simulink model "TxSteering_RxMVDR_4x4_HDL_IQ"  (R2020a)
settings: Solver=FixedStepDiscrete  StartTime=0.0  StopTime=stoptime*0 + inf  RelTol=1e-3
PreLoadFcn:
  | load('iq_bus_obj.mat');
  | model_init
InitFcn:
  | model_init
model workspace (MAT data in the model file):
  socvcb = containers.Map
  socvcb.serialization.keys = {}
  socvcb.serialization.values = {}
  socvcb.serialization.uniformity = 0
  socvcb.serialization.keyType = 'double'
  socvcb.serialization.valueType = 'any'
values from neighbouring files (symbols this model uses):
  BackSubstitutePrototype = fi(0, matrixdivbacksub_dt)    [model_init.m]
  DataSampleRate = ConverterSampleRate/DecimInterpFactor    (= 245760000)    [model_init.m]
  fc = ConverterSampleRate/4    (= 491520000)    [model_init.m]
  FPGAClkRate = DataSampleRate/VectorSamplingFactor    (= 245760000)    [model_init.m]
  matrixDivDelay = NumberOfCORDICIterations*10 + 86    [model_init.m]
  movavg_bitshift = nextpow2(sqrt(windowSize))    [model_init.m]
  mvdrPipelineDelay = covMatDelay+movAvgDelay+matrixDivDelay+normResponseDelay    [model_init.m]
  NCO_bits = 14    [model_init.m]
  numArrayElements = 4    [model_init.m]
  NumberOfCORDICIterations = matrixdivin_dt.WordLength - 1    [model_init.m]
  S2MM_frame_size = FrameSize*4    (= 40000)    [host_io_init.m]    (also in model_init.m = 1000)
  windowSize = 1024    [model_init.m]
undefined symbols (not defined in the file or in its folder): Fo, Fs, N, physconst
libraries: hdlsllib x268, simulink x53, dspsolvers x1, embreciprocals x1, dsphdlsigops x1
(part 1 of 12)
settings Model: DataTypeOverride=Off  Creator=mfornero  LastModifiedBy=tmealey
settings DataIOCC: SaveOutput=off  SaveTime=off  ReturnWorkspaceOutputs=off
settings OptimizationCC: BlockReduction=off  ConditionallyExecuteInputs=off  DefaultParameterBehavior=Inlined  LifeSpan=inf
settings DebuggingCC: AlgebraicLoopMsg=error  SingleTaskRateTransMsg=error  ParameterPrecisionLossMsg=none  PregeneratedLibrarySubsystemCodeDiagnostic=none  StrictBusMsg=ErrorOnBusTreatedAsVector  SFUnexpectedBacktrackingDiag=warning  SFNoUnconditionalDefaultTransitionDiag=warning  SFExecutionAtInitializationDiag=none  ArithmeticOperatorsInVariantConditions=warning
settings HardwareCC: ProdBitPerPointer=32  ProdBitPerSizeT=32  ProdBitPerPtrDiffT=32  ProdLargestAtomicFloat=None  ProdIntDivRoundTo=Undefined  ProdEndianess=Unspecified  ProdWordSize=32  ProdHWDeviceType=ASIC/FPGA->ASIC/FPGA  ProdEqTarget=off
settings SFSimCC: SimUseLocalCustomCode=off  CustomCodeUndefinedFunction=UseInterfaceOnly
settings RTWCC: RTWUseLocalCustomCode=off
settings CodeAppCC: StateflowObjectComments=on
settings GRTTargetCC: TargetLangStandard=C89/C90 (ANSI)
settings ConfigComp: CovMetricSettings=dw  CovHtmlReporting=on  CovSaveCumulativeToWorkspaceVar=on  CovSaveSingleToWorkspaceVar=on  CovExternalEMLEnable=off

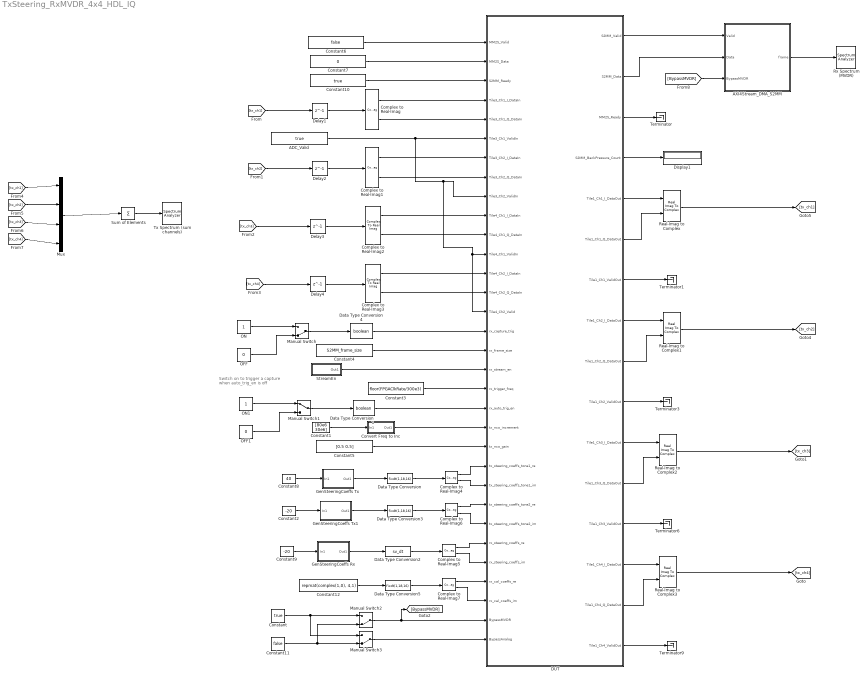
== system TxSteering_RxMVDR_4x4_HDL_IQ ==
  note: Switch on to trigger a capture
      | when auto_trig_en is off
  ADC_Valid : Constant  Value=true  SampleTime=-1
  AXI4Stream_DMA_S2MM : Subsystem
  Complex to Real-Imag{,1..7} (8 alike) : ComplexToRealImag
  Constant : Constant  Value=true  SampleTime=-1
  Constant1 : Constant  Value=[80e6 30e6]  OutDataTypeStr=double  SampleTime=-1
  Constant10 : Constant  Value=true  SampleTime=-1
  Constant11 : Constant  Value=false  SampleTime=-1
  Constant12 : Constant  Value=repmat(complex(1,0), 4,1)  OutDataTypeStr=double  SampleTime=-1
  Constant2 : Constant  Value=-20  OutDataTypeStr=double  SampleTime=-1
  Constant3 : Constant  Value=floor(FPGAClkRate/300e3)  OutDataTypeStr=uint32  SampleTime=-1
  Constant4 : Constant  Value=S2MM_frame_size  OutDataTypeStr=uint32  SampleTime=-1
  Constant5 : Constant  Value=[0.5 0.5]  OutDataTypeStr=fixdt(1,NCO_gain_bits,NCO_gain_bits-1)  SampleTime=-1
  Constant6 : Constant  Value=false  SampleTime=-1
  Constant7 : Constant  Value=0  OutDataTypeStr=fixdt(0,128,0)  SampleTime=-1
  Constant8 : Constant  Value=40  OutDataTypeStr=double  SampleTime=-1
  Constant9 : Constant  Value=-20  OutDataTypeStr=double  SampleTime=-1
  Convert Freq to Inc : Subsystem
  DUT : Subsystem  TreatAsAtomicUnit=on
  Data Type Conversion : DataTypeConversion  OutDataTypeStr=fixdt(1,18,16)
  Data Type Conversion1 : DataTypeConversion  OutDataTypeStr=boolean
  Data Type Conversion2 : DataTypeConversion  OutDataTypeStr=sv_dt
  Data Type Conversion3 : DataTypeConversion  OutDataTypeStr=fixdt(1,18,16)
  Data Type Conversion4 : DataTypeConversion  OutDataTypeStr=boolean
  Data Type Conversion5 : DataTypeConversion  OutDataTypeStr=fixdt(1,18,16)
  Delay{1..4} (4 alike) : Delay  DelayLength=1
  Display1 : Display
  GenSteeringCoeffs Rx : Subsystem
  GenSteeringCoeffs Tx : Subsystem
  GenSteeringCoeffs Tx1 : Subsystem
  Manual Switch : ManualSwitch  CurrentSetting=0
  Manual Switch1 : ManualSwitch
  Manual Switch2 : ManualSwitch  CurrentSetting=0
  Manual Switch3 : ManualSwitch  CurrentSetting=0
  Mux : Mux
  OFF : Constant  Value=0  OutDataTypeStr=boolean  SampleTime=-1
  OFF1 : Constant  Value=0  OutDataTypeStr=boolean  SampleTime=-1
  ON : Constant  OutDataTypeStr=boolean  SampleTime=-1
  ON1 : Constant  OutDataTypeStr=boolean  SampleTime=-1
  Real-Imag to Complex{,1..3} (4 alike) : RealImagToComplex
  Rx Spectrum (MVDR) : SpectrumAnalyzer
  StreamEn : Subsystem
  Sum of Elements : Sum  Inputs=+
  Terminator{,1,3,6,9} (5 alike) : Terminator
  Tx Spectrum (sum channels) : SpectrumAnalyzer
  wires:
  Real-Imag to Complex/1 -> [tx_ch1]
  DUT/2(S2MM_Data) -> AXI4Stream_DMA_S2MM/2(Data)
  Complex to Real-Imag3/2 -> DUT/14(Tile4_Ch2_Q_DataIn)
  Real-Imag to Complex2/1 -> [tx_ch3]
  Complex to Real-Imag4/2 -> DUT/24(tx_steering_coeffs_tone1_im)
  Real-Imag to Complex3/1 -> [tx_ch4]
  Manual Switch3/1 -> DUT/32(BypassAnalog)
  DUT/4(S2MM_BackPressure_Count) -> Display1/1
  Sum of Elements/1 -> Tx Spectrum (sum channels)/1
  Manual Switch2/1 -> [BypassMVDR], DUT/31(BypassMVDR)
  GenSteeringCoeffs Rx/1(Out1) -> Data Type Conversion2/1
  Complex to Real-Imag5/2 -> DUT/28(rx_steering_coeffs_im)
  Real-Imag to Complex1/1 -> [tx_ch2]
  Complex to Real-Imag6/2 -> DUT/26(tx_steering_coeffs_tone2_im)
  Complex to Real-Imag6/1 -> DUT/25(tx_steering_coeffs_tone2_re)
  Complex to Real-Imag5/1 -> DUT/27(rx_steering_coeffs_re)
  Constant2/1 -> GenSteeringCoeffs Tx1/1(In1)
  Convert Freq to Inc/1(Out1) -> DUT/21(tx_nco_increment)
  GenSteeringCoeffs Tx1/1(Out1) -> Data Type Conversion3/1
  Constant7/1 -> DUT/2(MM2S_Data)
  Data Type Conversion3/1 -> Complex to Real-Imag6/1
  [tx_ch4] -> Mux/4
  [tx_ch3] -> Mux/3
  Constant1/1 -> Convert Freq to Inc/1(In1)
  [tx_ch1] -> Mux/1
  [tx_ch2] -> Mux/2
  DUT/7(Tile1_Ch1_ValidOut) -> Terminator1/1
  Mux/1 -> Sum of Elements/1
  AXI4Stream_DMA_S2MM/1(frame) -> Rx Spectrum (MVDR)/1
  DUT/12(Tile1_Ch3_Q_DataOut) -> Real-Imag to Complex2/2
  Constant9/1 -> GenSteeringCoeffs Rx/1(In1)
  Complex to Real-Imag4/1 -> DUT/23(tx_steering_coeffs_tone1_re)
  Data Type Conversion2/1 -> Complex to Real-Imag5/1
  GenSteeringCoeffs Tx/1(Out1) -> Data Type Conversion/1
  Data Type Conversion/1 -> Complex to Real-Imag4/1
  Delay3/1 -> Complex to Real-Imag2/1
  Constant8/1 -> GenSteeringCoeffs Tx/1(In1)
  Constant5/1 -> DUT/22(tx_nco_gain)
  Constant6/1 -> DUT/1(MM2S_Valid)
  DUT/16(Tile1_Ch4_ValidOut) -> Terminator9/1
  Delay4/1 -> Complex to Real-Imag3/1
  [tx_ch4] -> Delay4/1
  Complex to Real-Imag1/1 -> DUT/7(Tile3_Ch2_I_DataIn)
  Complex to Real-Imag3/1 -> DUT/13(Tile4_Ch2_I_DataIn)
  Complex to Real-Imag2/2 -> DUT/11(Tile4_Ch1_Q_DataIn)
  Delay2/1 -> Complex to Real-Imag1/1
  Complex to Real-Imag2/1 -> DUT/10(Tile4_Ch1_I_DataIn)
  [tx_ch3] -> Delay3/1
  [tx_ch2] -> Delay2/1
  Complex to Real-Imag1/2 -> DUT/8(Tile3_Ch2_Q_DataIn)
  [tx_ch1] -> Delay1/1
  DUT/15(Tile1_Ch4_Q_DataOut) -> Real-Imag to Complex3/2
  DUT/14(Tile1_Ch4_I_DataOut) -> Real-Imag to Complex3/1
  DUT/10(Tile1_Ch2_ValidOut) -> Terminator3/1
  DUT/13(Tile1_Ch3_ValidOut) -> Terminator6/1
  DUT/11(Tile1_Ch3_I_DataOut) -> Real-Imag to Complex2/1
  Delay1/1 -> Complex to Real-Imag/1
  DUT/8(Tile1_Ch2_I_DataOut) -> Real-Imag to Complex1/1
  DUT/9(Tile1_Ch2_Q_DataOut) -> Real-Imag to Complex1/2
  DUT/5(Tile1_Ch1_I_DataOut) -> Real-Imag to Complex/1
  DUT/6(Tile1_Ch1_Q_DataOut) -> Real-Imag to Complex/2
  Complex to Real-Imag/2 -> DUT/5(Tile3_Ch1_Q_DataIn)
  Complex to Real-Imag/1 -> DUT/4("Tile3_Ch1_I_DataIn ")
  Constant10/1 -> DUT/3(S2MM_Ready)
  DUT/3(MM2S_Ready) -> Terminator/1
  DUT/1(S2MM_Valid) -> AXI4Stream_DMA_S2MM/1(Valid)
  Manual Switch1/1 -> Data Type Conversion1/1
  ON1/1 -> Manual Switch1/1
  OFF1/1 -> Manual Switch1/2
  Data Type Conversion1/1 -> DUT/20(rx_auto_trig_en)
  Constant3/1 -> DUT/19(rx_trigger_freq)
  StreamEn/1(Out1) -> DUT/18(rx_stream_en)
  OFF/1 -> Manual Switch/2
  ON/1 -> Manual Switch/1
  Manual Switch/1 -> Data Type Conversion4/1
  Constant4/1 -> DUT/17(rx_frame_size)
  Data Type Conversion4/1 -> DUT/16(rx_capture_trig)
  ADC_Valid/1 -> DUT/6(Tile3_Ch1_ValidIn), DUT/15(Tile4_Ch2_Valid), DUT/12(Tile4_Ch1_ValidIn), DUT/9(Tile3_Ch2_ValidIn)
  Constant/1 -> Manual Switch3/1, Manual Switch2/1
  Constant11/1 -> Manual Switch2/2, Manual Switch3/2
  [BypassMVDR] -> AXI4Stream_DMA_S2MM/3(BypassMVDR)
  Data Type Conversion5/1 -> Complex to Real-Imag7/1
  Complex to Real-Imag7/1 -> DUT/29(rx_cal_coeffs_re)
  Complex to Real-Imag7/2 -> DUT/30(rx_cal_coeffs_im)
  Constant12/1 -> Data Type Conversion5/1

== system TxSteering_RxMVDR_4x4_HDL_IQ/AXI4Stream_DMA_S2MM ==
  Valid : Inport
  Data : Inport  Port=2
  BypassMVDR : Inport  Port=3
  Display : Display
  Display1 : Display
  ForCalibration : Subsystem
  HDL Counter : hdlsllib/Sources/HDL Counter  CountType=Free running  CountInit=0  CountStep=1  CountMax=25  CountFromType=Initial value  CountFrom=0  CountResetPort=off  CountLoadPort=off  CountEnbPort=on  CountDirPort=off  CountDataType=Unsigned  CountWordLen=32  CountFracLen=0  CountSampTime=1
  HDL Counter1 : hdlsllib/Sources/HDL Counter  CountType=Free running  CountInit=0  CountStep=1  CountMax=25  CountFromType=Initial value  CountFrom=0  CountResetPort=off  CountLoadPort=off  CountEnbPort=on  CountDirPort=off  CountDataType=Unsigned  CountWordLen=32  CountFracLen=0  CountSampTime=1
  Logical Operator : Logic  AllPortsSameDT=off  OutDataTypeStr=boolean
  ProcessDataFrame : Subsystem
  "S2MM DMA plant " : Subsystem  mask{FRAME_SIZE=S2MM_frame_size}
      mask prompts: FRAME_SIZE "Frame size:"
  frame : Outport
  wires:
  "S2MM DMA plant "/2(frame_valid) -> HDL Counter1/1, Logical Operator/1, ProcessDataFrame/Enable
  Data/1 -> "S2MM DMA plant "/1(data_in)
  Valid/1 -> HDL Counter/1, "S2MM DMA plant "/2(valid_in)
  ProcessDataFrame/1(Out1) -> frame/1
  BypassMVDR/1 -> Logical Operator/2
  Logical Operator/1 -> ForCalibration/Enable
  "S2MM DMA plant "/1(frame_data) -> ProcessDataFrame/1(In1), ForCalibration/1(In1)
  HDL Counter/1 -> Display/1
  HDL Counter1/1 -> Display1/1

== system TxSteering_RxMVDR_4x4_HDL_IQ/Convert Freq to Inc ==
  In1 : Inport
  Data Type Conversion : DataTypeConversion  OutDataTypeStr=fixdt(0,NCO_bits,0)
  Floor : Rounding
  Gain : Gain  Gain=2^NCO_bits/DataSampleRate
  Out1 : Outport
  wires:
  In1/1 -> Gain/1
  Gain/1 -> Floor/1
  Floor/1 -> Data Type Conversion/1
  Data Type Conversion/1 -> Out1/1

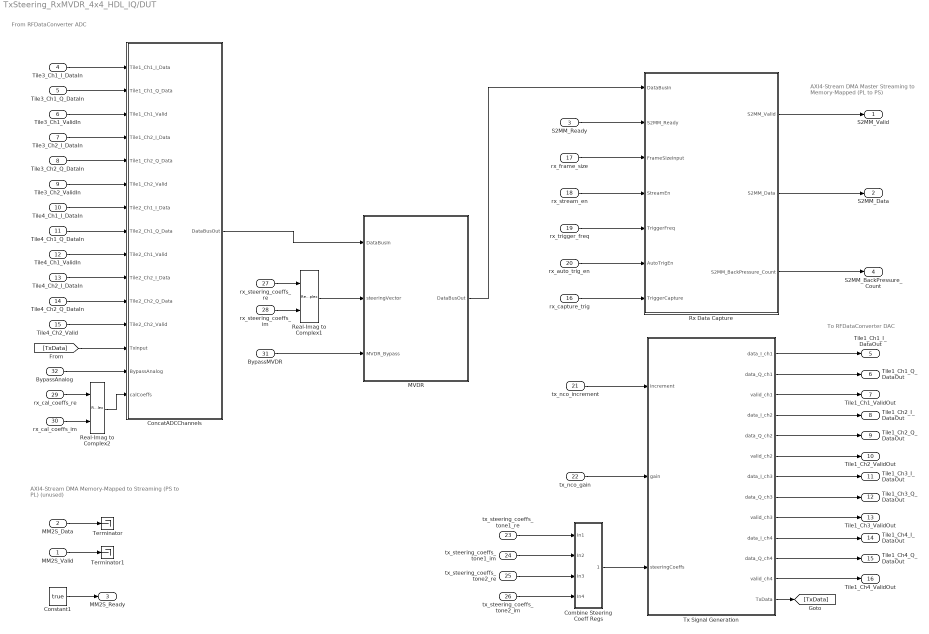
== system TxSteering_RxMVDR_4x4_HDL_IQ/DUT ==
  note: AXI4-Stream DMA Master
      | Streaming to Memory-Mapped (PL to PS)
  note: AXI4-Stream DMA
      | Memory-Mapped to Streaming (PS to PL)
      | (unused)
  note: From RFDataConverter ADC
  note: To RFDataConverter DAC
  MM2S_Valid : Inport
  MM2S_Data : Inport  Port=2
  S2MM_Ready : Inport  Port=3
  "Tile3_Ch1_I_DataIn " : Inport  Port=4
  Tile3_Ch1_Q_DataIn : Inport  Port=5
  Tile3_Ch1_ValidIn : Inport  Port=6
  Tile3_Ch2_I_DataIn : Inport  Port=7
  Tile3_Ch2_Q_DataIn : Inport  Port=8
  Tile3_Ch2_ValidIn : Inport  Port=9
  Tile4_Ch1_I_DataIn : Inport  Port=10
  Tile4_Ch1_Q_DataIn : Inport  Port=11
  Tile4_Ch1_ValidIn : Inport  Port=12
  Tile4_Ch2_I_DataIn : Inport  Port=13
  Tile4_Ch2_Q_DataIn : Inport  Port=14
  Tile4_Ch2_Valid : Inport  Port=15
  rx_capture_trig : Inport  Port=16
  rx_frame_size : Inport  Port=17
  rx_stream_en : Inport  Port=18
  rx_trigger_freq : Inport  Port=19
  rx_auto_trig_en : Inport  Port=20
  tx_nco_increment : Inport  Port=21  OutDataTypeStr=fixdt(0,NCO_bits,0)
  tx_nco_gain : Inport  Port=22  OutDataTypeStr=fixdt(1,NCO_gain_bits,NCO_gain_bits-1)
  tx_steering_coeffs_tone1_re : Inport  Port=23  PortDimensions=NumChan
  tx_steering_coeffs_tone1_im : Inport  Port=24  PortDimensions=NumChan
  tx_steering_coeffs_tone2_re : Inport  Port=25  PortDimensions=NumChan
  tx_steering_coeffs_tone2_im : Inport  Port=26  PortDimensions=NumChan
  rx_steering_coeffs_re : Inport  Port=27  PortDimensions=NumChan
  rx_steering_coeffs_im : Inport  Port=28  PortDimensions=NumChan
  rx_cal_coeffs_re : Inport  Port=29  PortDimensions=NumChan
  rx_cal_coeffs_im : Inport  Port=30  PortDimensions=NumChan
  BypassMVDR : Inport  Port=31
  BypassAnalog : Inport  Port=32
  Combine Steering Coeff Regs : Subsystem
  ConcatADCChannels : Subsystem
  Constant1 : Constant  Value=true  OutDataTypeStr=boolean  SampleTime=-1
  MVDR : Subsystem
  Real-Imag to Complex1 : RealImagToComplex
  Real-Imag to Complex2 : RealImagToComplex
  Rx Data Capture : Subsystem
  Terminator : Terminator
  Terminator1 : Terminator
  Tx Signal Generation : Subsystem
  S2MM_Valid : Outport  VectorParamsAs1DForOutWhenUnconnected=off
  S2MM_Data : Outport  Port=2  VectorParamsAs1DForOutWhenUnconnected=off
  MM2S_Ready : Outport  Port=3  VectorParamsAs1DForOutWhenUnconnected=off
  S2MM_BackPressure_Count : Outport  Port=4  VectorParamsAs1DForOutWhenUnconnected=off
  Tile1_Ch1_I_DataOut : Outport  Port=5  VectorParamsAs1DForOutWhenUnconnected=off
  Tile1_Ch1_Q_DataOut : Outport  Port=6  VectorParamsAs1DForOutWhenUnconnected=off
  Tile1_Ch1_ValidOut : Outport  Port=7  VectorParamsAs1DForOutWhenUnconnected=off
  Tile1_Ch2_I_DataOut : Outport  Port=8  VectorParamsAs1DForOutWhenUnconnected=off
  Tile1_Ch2_Q_DataOut : Outport  Port=9  VectorParamsAs1DForOutWhenUnconnected=off
  Tile1_Ch2_ValidOut : Outport  Port=10  VectorParamsAs1DForOutWhenUnconnected=off
  Tile1_Ch3_I_DataOut : Outport  Port=11  VectorParamsAs1DForOutWhenUnconnected=off
  Tile1_Ch3_Q_DataOut : Outport  Port=12  VectorParamsAs1DForOutWhenUnconnected=off
  Tile1_Ch3_ValidOut : Outport  Port=13  VectorParamsAs1DForOutWhenUnconnected=off
  Tile1_Ch4_I_DataOut : Outport  Port=14  VectorParamsAs1DForOutWhenUnconnected=off
  Tile1_Ch4_Q_DataOut : Outport  Port=15  VectorParamsAs1DForOutWhenUnconnected=off
  Tile1_Ch4_ValidOut : Outport  Port=16  VectorParamsAs1DForOutWhenUnconnected=off
  wires:
  Constant1/1 -> MM2S_Ready/1
  S2MM_Ready/1 -> Rx Data Capture/2(S2MM_Ready)
  rx_frame_size/1 -> Rx Data Capture/3(FrameSizeInput)
  rx_stream_en/1 -> Rx Data Capture/4(StreamEn)
  rx_trigger_freq/1 -> Rx Data Capture/5(TriggerFreq)
  rx_auto_trig_en/1 -> Rx Data Capture/6(AutoTrigEn)
  rx_capture_trig/1 -> Rx Data Capture/7(TriggerCapture)
  Rx Data Capture/1(S2MM_Valid) -> S2MM_Valid/1
  Rx Data Capture/2(S2MM_Data) -> S2MM_Data/1
  Rx Data Capture/3(S2MM_BackPressure_Count) -> S2MM_BackPressure_Count/1
  "Tile3_Ch1_I_DataIn "/1 -> ConcatADCChannels/1("Tile1_Ch1_I_Data ")
  Tile3_Ch1_ValidIn/1 -> ConcatADCChannels/3(Tile1_Ch1_Valid)
  Tile3_Ch1_Q_DataIn/1 -> ConcatADCChannels/2(Tile1_Ch1_Q_Data)
  Tile3_Ch2_I_DataIn/1 -> ConcatADCChannels/4(Tile1_Ch2_I_Data)
  Tile3_Ch2_ValidIn/1 -> ConcatADCChannels/6(Tile1_Ch2_Valid)
  Tile3_Ch2_Q_DataIn/1 -> ConcatADCChannels/5(Tile1_Ch2_Q_Data)
  Tile4_Ch1_I_DataIn/1 -> ConcatADCChannels/7(Tile2_Ch1_I_Data)
  Tile4_Ch1_ValidIn/1 -> ConcatADCChannels/9(Tile2_Ch1_Valid)
  Tile4_Ch1_Q_DataIn/1 -> ConcatADCChannels/8(Tile2_Ch1_Q_Data)
  Tile4_Ch2_I_DataIn/1 -> ConcatADCChannels/10(Tile2_Ch2_I_Data)
  Tile4_Ch2_Valid/1 -> ConcatADCChannels/12(Tile2_Ch2_Valid)
  Tile4_Ch2_Q_DataIn/1 -> ConcatADCChannels/11(Tile2_Ch2_Q_Data)
  MM2S_Data/1 -> Terminator/1
  MM2S_Valid/1 -> Terminator1/1
  Tx Signal Generation/1(data_I_ch1) -> Tile1_Ch1_I_DataOut/1
  Tx Signal Generation/2(data_Q_ch1) -> Tile1_Ch1_Q_DataOut/1
  tx_nco_increment/1 -> Tx Signal Generation/1(increment)
  tx_nco_gain/1 -> Tx Signal Generation/2(gain)
  Tx Signal Generation/3(valid_ch1) -> Tile1_Ch1_ValidOut/1
  Tx Signal Generation/4(data_I_ch2) -> Tile1_Ch2_I_DataOut/1
  Tx Signal Generation/5(data_Q_ch2) -> Tile1_Ch2_Q_DataOut/1
  Tx Signal Generation/6(valid_ch2) -> Tile1_Ch2_ValidOut/1
  Tx Signal Generation/7(data_I_ch3) -> Tile1_Ch3_I_DataOut/1
  Tx Signal Generation/8(data_Q_ch3) -> Tile1_Ch3_Q_DataOut/1
  Tx Signal Generation/9(valid_ch3) -> Tile1_Ch3_ValidOut/1
  Tx Signal Generation/10(data_I_ch4) -> Tile1_Ch4_I_DataOut/1
  Tx Signal Generation/11(data_Q_ch4) -> Tile1_Ch4_Q_DataOut/1
  Tx Signal Generation/12(valid_ch4) -> Tile1_Ch4_ValidOut/1
  rx_steering_coeffs_im/1 -> Real-Imag to Complex1/2
  Real-Imag to Complex1/1 -> MVDR/2(steeringVector)
  rx_steering_coeffs_re/1 -> Real-Imag to Complex1/1
  ConcatADCChannels/1(DataBusOut) -> MVDR/1(DataBusIn)
  tx_steering_coeffs_tone1_re/1 -> Combine Steering Coeff Regs/1(In1)
  tx_steering_coeffs_tone1_im/1 -> Combine Steering Coeff Regs/2(In2)
  tx_steering_coeffs_tone2_re/1 -> Combine Steering Coeff Regs/3(In3)
  tx_steering_coeffs_tone2_im/1 -> Combine Steering Coeff Regs/4(In4)
  Combine Steering Coeff Regs/1(Out1) -> Tx Signal Generation/3(steeringCoeffs)
  MVDR/1(DataBusOut) -> Rx Data Capture/1(DataBusIn)
  Tx Signal Generation/13(TxData) -> [TxData]
  [TxData] -> ConcatADCChannels/13(TxInput)
  BypassMVDR/1 -> MVDR/3(MVDR_Bypass)
  BypassAnalog/1 -> ConcatADCChannels/14(BypassAnalog)
  rx_cal_coeffs_re/1 -> Real-Imag to Complex2/1
  rx_cal_coeffs_im/1 -> Real-Imag to Complex2/2
  Real-Imag to Complex2/1 -> ConcatADCChannels/15(calCoeffs)

== system TxSteering_RxMVDR_4x4_HDL_IQ/GenSteeringCoeffs Rx ==
  In1 : Inport
  Constant : Constant  Value=fc  SampleTime=-1
  Constant9 : Constant  Value=0  OutDataTypeStr=double  SampleTime=-1
  MATLAB System1 : MATLABSystem  System=phased.SteeringVector  PropagationSpeed=physconst( 'LightSpeed' )  IncludeElementResponse=off  NumPhaseShifterBits=0  EnablePolarization=off  SimulateUsing=Interpreted execution  SensorArray=sensorArray
      mask Type: phased.SteeringVector
      mask Display:
      | disp(['Steering' char(10) 'Vector']);
      | port_label('input',1,'Freq');
      | port_label('input',2,'Ang');
  Vector Concatenate : Concatenate  Mode=Multidimensional array
  Out1 : Outport
  wires:
  Vector Concatenate/1 -> MATLAB System1/2
  Constant/1 -> MATLAB System1/1
  In1/1 -> Vector Concatenate/1
  Constant9/1 -> Vector Concatenate/2
  MATLAB System1/1 -> Out1/1

== system TxSteering_RxMVDR_4x4_HDL_IQ/GenSteeringCoeffs Tx ==
  In1 : Inport
  Constant : Constant  Value=fc  SampleTime=-1
  Constant9 : Constant  Value=0  OutDataTypeStr=double  SampleTime=-1
  MATLAB System1 : MATLABSystem  System=phased.SteeringVector  PropagationSpeed=physconst( 'LightSpeed' )  IncludeElementResponse=off  NumPhaseShifterBits=0  EnablePolarization=off  SimulateUsing=Interpreted execution  SensorArray=sensorArray
      mask Type: phased.SteeringVector
      mask Display:
      | disp(['Steering' char(10) 'Vector']);
      | port_label('input',1,'Freq');
      | port_label('input',2,'Ang');
  Vector Concatenate : Concatenate  Mode=Multidimensional array
  Out1 : Outport
  wires:
  MATLAB System1/1 -> Out1/1
  Constant9/1 -> Vector Concatenate/2
  In1/1 -> Vector Concatenate/1
  Constant/1 -> MATLAB System1/1
  Vector Concatenate/1 -> MATLAB System1/2

== system TxSteering_RxMVDR_4x4_HDL_IQ/GenSteeringCoeffs Tx1 ==
  In1 : Inport
  Constant : Constant  Value=fc  SampleTime=-1
  Constant9 : Constant  Value=0  OutDataTypeStr=double  SampleTime=-1
  MATLAB System1 : MATLABSystem  System=phased.SteeringVector  PropagationSpeed=physconst( 'LightSpeed' )  IncludeElementResponse=off  NumPhaseShifterBits=0  EnablePolarization=off  SimulateUsing=Interpreted execution  SensorArray=sensorArray
      mask Type: phased.SteeringVector
      mask Display:
      | disp(['Steering' char(10) 'Vector']);
      | port_label('input',1,'Freq');
      | port_label('input',2,'Ang');
  Vector Concatenate : Concatenate  Mode=Multidimensional array
  Out1 : Outport
  wires:
  Vector Concatenate/1 -> MATLAB System1/2
  Constant/1 -> MATLAB System1/1
  In1/1 -> Vector Concatenate/1
  Constant9/1 -> Vector Concatenate/2
  MATLAB System1/1 -> Out1/1

== system TxSteering_RxMVDR_4x4_HDL_IQ/StreamEn ==
  Data Type Conversion1 : DataTypeConversion  OutDataTypeStr=boolean
  Manual Switch1 : ManualSwitch
  OFF : Constant  Value=0  OutDataTypeStr=boolean  SampleTime=-1
  ON : Constant  OutDataTypeStr=boolean  SampleTime=-1
  Out1 : Outport  VectorParamsAs1DForOutWhenUnconnected=off
  wires:
  Data Type Conversion1/1 -> Out1/1
  OFF/1 -> Manual Switch1/2
  ON/1 -> Manual Switch1/1
  Manual Switch1/1 -> Data Type Conversion1/1

== system TxSteering_RxMVDR_4x4_HDL_IQ/AXI4Stream_DMA_S2MM/ForCalibration ==
  In1 : Inport
  Enable : EnablePort
  Rx Spectrum (MVDR) : SpectrumAnalyzer
  Selector : Selector  NumberOfDimensions=2  InputPortWidth=3  IndexOptions=Select all,Index vector (dialog)  Indices=[1 3],1  OutputSizes=1,1
  Selector1 : Selector  NumberOfDimensions=2  InputPortWidth=3  IndexOptions=Select all,Index vector (dialog)  Indices=[1 3],2  OutputSizes=1,1
  Selector2 : Selector  NumberOfDimensions=2  InputPortWidth=3  IndexOptions=Select all,Index vector (dialog)  Indices=[1 3],3  OutputSizes=1,1
  Selector3 : Selector  NumberOfDimensions=2  InputPortWidth=3  IndexOptions=Select all,Index vector (dialog)  Indices=[1 3],4  OutputSizes=1,1
  Time Scope : Scope  NumInputPorts=4
  Unpack Complex : Subsystem
  wires:
  In1/1 -> Unpack Complex/1(In1)
  Unpack Complex/1(Out1) -> Selector3/1, Selector2/1, Selector1/1, Selector/1
  Selector1/1 -> Time Scope/2
  Selector/1 -> Time Scope/1
  Selector2/1 -> Time Scope/3
  Selector3/1 -> Rx Spectrum (MVDR)/1, Time Scope/4

== system TxSteering_RxMVDR_4x4_HDL_IQ/AXI4Stream_DMA_S2MM/ProcessDataFrame ==
  In1 : Inport
  Enable : EnablePort
  Data Type Conversion5 : DataTypeConversion  OutDataTypeStr=fixdt(1,64,0)  ConvertRealWorld=Stored Integer (SI)
  Unpack Complex : Subsystem
  Out1 : Outport
  wires:
  In1/1 -> Data Type Conversion5/1
  Unpack Complex/1(Out1) -> Out1/1
  Data Type Conversion5/1 -> Unpack Complex/1(In1)

== system TxSteering_RxMVDR_4x4_HDL_IQ/AXI4Stream_DMA_S2MM/S2MM DMA plant  ==
  data_in : Inport
  valid_in : Inport  Port=2
  MATLAB Function1 : MATLAB Function  TreatAsAtomicUnit=on
  frame_data : Outport
  frame_valid : Outport  Port=2
  wires:
  valid_in/1 -> MATLAB Function1/2(valid_i)
  MATLAB Function1/1(data_o) -> frame_data/1
  MATLAB Function1/2(valid_o) -> frame_valid/1
  data_in/1 -> MATLAB Function1/1(data_i)

== system TxSteering_RxMVDR_4x4_HDL_IQ/DUT/Combine Steering Coeff Regs ==
  In1 : Inport
  In2 : Inport  Port=2
  In3 : Inport  Port=3
  In4 : Inport  Port=4
  Real-Imag to Complex : RealImagToComplex
  Real-Imag to Complex2 : RealImagToComplex
  Vector Concatenate : Concatenate
  Out1 : Outport
  wires:
  In1/1 -> Real-Imag to Complex/1
  In2/1 -> Real-Imag to Complex/2
  In4/1 -> Real-Imag to Complex2/2
  In3/1 -> Real-Imag to Complex2/1
  Real-Imag to Complex/1 -> Vector Concatenate/1
  Real-Imag to Complex2/1 -> Vector Concatenate/2
  Vector Concatenate/1 -> Out1/1

== system TxSteering_RxMVDR_4x4_HDL_IQ/DUT/ConcatADCChannels ==
  "Tile1_Ch1_I_Data " : Inport
  Tile1_Ch1_Q_Data : Inport  Port=2
  Tile1_Ch1_Valid : Inport  Port=3
  Tile1_Ch2_I_Data : Inport  Port=4
  Tile1_Ch2_Q_Data : Inport  Port=5
  Tile1_Ch2_Valid : Inport  Port=6
  Tile2_Ch1_I_Data : Inport  Port=7
  Tile2_Ch1_Q_Data : Inport  Port=8
  Tile2_Ch1_Valid : Inport  Port=9
  Tile2_Ch2_I_Data : Inport  Port=10
  Tile2_Ch2_Q_Data : Inport  Port=11
  Tile2_Ch2_Valid : Inport  Port=12
  TxInput : Inport  Port=13
  BypassAnalog : Inport  Port=14
  calCoeffs : Inport  Port=15
  Apply Calibration Coefficients : Subsystem
  Data Type Conversion : DataTypeConversion  OutDataTypeStr=input_dt  ConvertRealWorld=Stored Integer (SI)
  Delay1 : Delay  DelayLength=1
  Delay2 : Delay  DelayLength=1
  Real-Imag to Complex{,1..3} (4 alike) : RealImagToComplex
  Switch : Switch  Criteria=u2 > Threshold
  Terminator : Terminator
  Terminator3 : Terminator
  Terminator5 : Terminator
  To Data Bus : Subsystem  mask(To Data Bus){dummy=0}
      mask help: Create a streaming Data Bus from Data and Valid signals.
      mask Display:
      | port_label('input',1,'data');
      | port_label('input',2,'valid');
  Vector Concatenate : Concatenate  NumInputs=4  Mode=Multidimensional array  ConcatenateDimension=2
  DataBusOut : Outport  VectorParamsAs1DForOutWhenUnconnected=off
  wires:
  Tile1_Ch2_Valid/1 -> Terminator/1
  Tile2_Ch1_Valid/1 -> Terminator3/1
  Tile2_Ch2_Valid/1 -> Terminator5/1
  Real-Imag to Complex/1 -> Vector Concatenate/1
  Real-Imag to Complex1/1 -> Vector Concatenate/2
  Real-Imag to Complex2/1 -> Vector Concatenate/3
  Real-Imag to Complex3/1 -> Vector Concatenate/4
  Vector Concatenate/1 -> Data Type Conversion/1
  To Data Bus/1(bus) -> Delay2/1
  "Tile1_Ch1_I_Data "/1 -> Real-Imag to Complex/1
  Tile1_Ch1_Q_Data/1 -> Real-Imag to Complex/2
  Tile1_Ch2_I_Data/1 -> Real-Imag to Complex1/1
  Tile1_Ch2_Q_Data/1 -> Real-Imag to Complex1/2
  Tile2_Ch1_I_Data/1 -> Real-Imag to Complex2/1
  Tile2_Ch1_Q_Data/1 -> Real-Imag to Complex2/2
  Tile2_Ch2_I_Data/1 -> Real-Imag to Complex3/1
  Tile2_Ch2_Q_Data/1 -> Real-Imag to Complex3/2
  TxInput/1 -> Switch/1
  Switch/1 -> Delay1/1
  BypassAnalog/1 -> Switch/2
  Delay1/1 -> DataBusOut/1
  Delay2/1 -> Switch/3
  Data Type Conversion/1 -> Apply Calibration Coefficients/1(dataIn)
  Apply Calibration Coefficients/1(dataOut) -> To Data Bus/1(data)
  Apply Calibration Coefficients/2(validOut) -> To Data Bus/2(valid)
  calCoeffs/1 -> Apply Calibration Coefficients/3(coeffIn)
  Tile1_Ch1_Valid/1 -> Apply Calibration Coefficients/2(validIn)

== system TxSteering_RxMVDR_4x4_HDL_IQ/DUT/MVDR ==
  DataBusIn : Inport
  steeringVector : Inport  Port=2
  MVDR_Bypass : Inport  Port=3
  Compute Weight Vector : Subsystem
  Delay5 : Delay  DelayLength=mvdrPipelineDelay
  Form Beam : Subsystem
  Form Covariance Matrix : Subsystem
  From Data Bus : Subsystem  mask(From Data Bus){dummy=0}
      mask help: Convert a streaming Data Bus to individual Data and Valid signals.
      mask Display:
      | port_label('output',1,'data');
      | port_label('output',2,'valid');
  Moving Average : Subsystem
  Normalize Response : Subsystem
  Subsystem : Subsystem
  DataBusOut : Outport
  wires:
  Form Covariance Matrix/2(validOut) -> Moving Average/2(validIn)
  Compute Weight Vector/1(w) -> Normalize Response/1(wIn)
  steeringVector/1 -> Normalize Response/3(steeringVector), Compute Weight Vector/3(steeringVector)
  Form Covariance Matrix/1(dataOut) -> Moving Average/1(dataIn)
  DataBusIn/1 -> Delay5/1, Subsystem/2(Bypass_Input), From Data Bus/1(bus)
  Moving Average/1(dataOut) -> Compute Weight Vector/1(covarianceMatrix)
  Delay5/1 -> Form Beam/1(DataBusIn)
  Moving Average/2(validOut) -> Compute Weight Vector/2(validIn)
  From Data Bus/2(valid) -> Form Covariance Matrix/2(validIn)
  From Data Bus/1(data) -> Form Covariance Matrix/1(dataIn)
  Form Beam/1(DataBusOut) -> Subsystem/3(MVDR_Input)
  Subsystem/1(DataOut) -> DataBusOut/1
  MVDR_Bypass/1 -> Subsystem/1(BypassEn)
  Compute Weight Vector/2(validOut) -> Normalize Response/2(validIn)
  Normalize Response/1(wOut) -> Form Beam/2(w)

== system TxSteering_RxMVDR_4x4_HDL_IQ/DUT/Rx Data Capture ==
  Bus Element In : Inport  PortName=DataBusIn  Element=data
  Bus Element In1 : Inport  PortName=DataBusIn  Element=valid
  S2MM_Ready : Inport  Port=2
  FrameSizeInput : Inport  Port=3
  StreamEn : Inport  Port=4
  TriggerFreq : Inport  Port=5
  AutoTrigEn : Inport  Port=6
  TriggerCapture : Inport  Port=7
  AXI4-Lite Initial Value : Subsystem  mask(AXI4-Lite Initial Value){x0=uint32(floor(FPGAClkRate/2))}
      mask prompts: x0 "Initial value:"
      mask help: Set the initial value for an AXI4-Lite register.
      mask Display: fprintf('x0 = %g',x0);
  AutoTrigger : Subsystem
  Delay{2,4..6,25..26} (6 alike) : Delay  DelayLength=1
  EnableConsecutiveFrames : Subsystem
  HDL Counter : hdlsllib/Sources/HDL Counter  CountType=Free running  CountInit=0  CountStep=1  CountMax=25  CountFromType=Initial value  CountFrom=0  CountResetPort=off  CountLoadPort=off  CountEnbPort=on  CountDirPort=off  CountDataType=Unsigned  CountWordLen=32  CountFracLen=0  CountSampTime=1
  Logical Operator6 : Logic  Operator=NOT  IconShape=distinctive  AllPortsSameDT=off  OutDataTypeStr=boolean
  Signal Specification : SignalSpecification  SampleTime=1/FPGAClkRate
  "Stream FIFO " : Subsystem
  Switch : Switch  Criteria=u2 > Threshold
  Terminator : Terminator
  Terminator3 : Terminator
  S2MM_Valid : Outport  VectorParamsAs1DForOutWhenUnconnected=off
  S2MM_Data : Outport  Port=2  VectorParamsAs1DForOutWhenUnconnected=off
  S2MM_BackPressure_Count : Outport  Port=3  VectorParamsAs1DForOutWhenUnconnected=off
  wires:
  S2MM_Ready/1 -> Delay4/1
  Delay6/1 -> AutoTrigger/2(SW_en), "Stream FIFO "/5(StreamEn)
  Delay26/1 -> "Stream FIFO "/3(TValid)
  AutoTrigger/1(Trig) -> Switch/1  "Trig"
  TriggerCapture/1 -> Delay5/1
  FrameSizeInput/1 -> Delay2/1
  Delay4/1 -> "Stream FIFO "/1(TReady)
  StreamEn/1 -> Delay6/1
  Delay5/1 -> Switch/3
  "Stream FIFO "/5(AFull) -> HDL Counter/1, Logical Operator6/1  "AlmostFull"
  "Stream FIFO "/2(ValidOut) -> S2MM_Valid/1
  EnableConsecutiveFrames/1(DataCaptureEn) -> "Stream FIFO "/4(TriggerCapture)
  "Stream FIFO "/4(Full) -> Terminator3/1
  Logical Operator6/1 -> EnableConsecutiveFrames/3(BackPressureCounterEn)
  TriggerFreq/1 -> AXI4-Lite Initial Value/1(In1)
  AXI4-Lite Initial Value/1(Out1) -> AutoTrigger/1(MaxCount)
  "Stream FIFO "/3(Num) -> Terminator/1
  AutoTrigEn/1 -> Switch/2
  Delay25/1 -> Signal Specification/1
  Delay2/1 -> EnableConsecutiveFrames/2(ConsecFrames)
  Switch/1 -> EnableConsecutiveFrames/1(Trigger)  "TriggerInput"
  HDL Counter/1 -> S2MM_BackPressure_Count/1
  "Stream FIFO "/1(TDataOut) -> S2MM_Data/1
  Bus Element In1/1 -> Delay26/1
  Signal Specification/1 -> "Stream FIFO "/2(TData)
  Bus Element In/1 -> Delay25/1

== system TxSteering_RxMVDR_4x4_HDL_IQ/DUT/Tx Signal Generation ==
  increment : Inport
  gain : Inport  Port=2
  steeringCoeffs : Inport  Port=3
  Combine Channels : Subsystem
  Complex to Real-Imag : ComplexToRealImag
  ConcatADCChannels : Subsystem
  Delay : Delay  DelayLength=1
  Demux : Demux
  Demux1 : Demux
  Generate Steering Channels : Subsystem  TreatAsAtomicUnit=on
  data_I_ch1 : Outport
  data_Q_ch1 : Outport  Port=2
  valid_ch1 : Outport  Port=3
  data_I_ch2 : Outport  Port=4
  data_Q_ch2 : Outport  Port=5
  valid_ch2 : Outport  Port=6
  data_I_ch3 : Outport  Port=7
  data_Q_ch3 : Outport  Port=8
  valid_ch3 : Outport  Port=9
  data_I_ch4 : Outport  Port=10
  data_Q_ch4 : Outport  Port=11
  valid_ch4 : Outport  Port=12
  TxData : Outport  Port=13
  wires:
  Demux/1 -> data_I_ch1/1, ConcatADCChannels/1("Tile1_Ch1_I_Data ")
  Demux/4 -> data_I_ch4/1, ConcatADCChannels/7(Tile2_Ch2_I_Data)
  Demux/3 -> data_I_ch3/1, ConcatADCChannels/5(Tile2_Ch1_I_Data)
  Demux/2 -> ConcatADCChannels/3(Tile1_Ch2_I_Data), data_I_ch2/1
  Demux1/1 -> ConcatADCChannels/2(Tile1_Ch1_Q_Data), data_Q_ch1/1
  Demux1/2 -> ConcatADCChannels/4(Tile1_Ch2_Q_Data), data_Q_ch2/1
  Demux1/3 -> ConcatADCChannels/6(Tile2_Ch1_Q_Data), data_Q_ch3/1
  Demux1/4 -> ConcatADCChannels/8(Tile2_Ch2_Q_Data), data_Q_ch4/1
  Complex to Real-Imag/2 -> Demux1/1
  Complex to Real-Imag/1 -> Demux/1
  increment/1 -> Generate Steering Channels/1(increment)
  gain/1 -> Generate Steering Channels/2(gain)
  steeringCoeffs/1 -> Generate Steering Channels/3(steeringCoeffs)
  Combine Channels/2(validOut) -> ConcatADCChannels/9(Valid), valid_ch1/1, valid_ch4/1, valid_ch3/1, valid_ch2/1
  Generate Steering Channels/1(dataOut) -> Combine Channels/1(dataIn)
  Generate Steering Channels/2(validOut) -> Combine Channels/2(validIn)
  Combine Channels/1(dataOut) -> Complex to Real-Imag/1
  ConcatADCChannels/1(DataBusOut) -> Delay/1
  Delay/1 -> TxData/1

== system TxSteering_RxMVDR_4x4_HDL_IQ/AXI4Stream_DMA_S2MM/ForCalibration/Unpack Complex ==
  In1 : Inport
  Extract Bits2 : simulink/Logic and Bit Operations/Extract Bits  bitsToExtract=Lower half  numBits=8  bitIdxRange=[0 7]  outScalingMode=Treat bit field as an integer
  Extract Bits3 : simulink/Logic and Bit Operations/Extract Bits  bitsToExtract=Upper half  numBits=8  bitIdxRange=[0 7]  outScalingMode=Treat bit field as an integer
  For Each Subsystem : Subsystem  Commented=on  TreatAsAtomicUnit=on
  Real-Imag to Complex{1..4} (4 alike) : RealImagToComplex
  Subsystem : Subsystem
  Subsystem1 : Subsystem
  Vector Concatenate1 : Concatenate  NumInputs=4  Mode=Multidimensional array  ConcatenateDimension=2
  Out1 : Outport  VectorParamsAs1DForOutWhenUnconnected=off
  wires:
  In1/1 -> Extract Bits3/1, Extract Bits2/1
  Extract Bits2/1 -> Subsystem/1(In1)
  Extract Bits3/1 -> Subsystem1/1(In1)
  Subsystem/4(Out4) -> Real-Imag to Complex2/2
  Subsystem1/1(Out1) -> Real-Imag to Complex3/1
  Subsystem/3(Out3) -> Real-Imag to Complex2/1
  Subsystem1/2(Out2) -> Real-Imag to Complex3/2
  Subsystem/2(Out2) -> Real-Imag to Complex1/2
  Subsystem1/3(Out3) -> Real-Imag to Complex4/1
  Subsystem/1(Out1) -> Real-Imag to Complex1/1
  Subsystem1/4(Out4) -> Real-Imag to Complex4/2
  Real-Imag to Complex2/1 -> Vector Concatenate1/2
  Real-Imag to Complex1/1 -> Vector Concatenate1/1
  Real-Imag to Complex3/1 -> Vector Concatenate1/3
  Real-Imag to Complex4/1 -> Vector Concatenate1/4
  Vector Concatenate1/1 -> Out1/1

== system TxSteering_RxMVDR_4x4_HDL_IQ/AXI4Stream_DMA_S2MM/ProcessDataFrame/Unpack Complex ==
  In1 : Inport
  Data Type Conversion : DataTypeConversion  OutDataTypeStr=output_dt  ConvertRealWorld=Stored Integer (SI)
  Extract Bits : simulink/Logic and Bit Operations/Extract Bits  bitsToExtract=Upper half  numBits=8  bitIdxRange=[0 7]  outScalingMode=Treat bit field as an integer
  Extract Bits1 : simulink/Logic and Bit Operations/Extract Bits  bitsToExtract=Lower half  numBits=8  bitIdxRange=[0 7]  outScalingMode=Treat bit field as an integer
  Real-Imag to Complex : RealImagToComplex
  Out1 : Outport  VectorParamsAs1DForOutWhenUnconnected=off
  wires:
  Extract Bits/1 -> Real-Imag to Complex/2
  Extract Bits1/1 -> Real-Imag to Complex/1
  Data Type Conversion/1 -> Out1/1
  Real-Imag to Complex/1 -> Data Type Conversion/1
  In1/1 -> Extract Bits1/1, Extract Bits/1

== system TxSteering_RxMVDR_4x4_HDL_IQ/DUT/ConcatADCChannels/Apply Calibration Coefficients ==
  dataIn : Inport
  validIn : Inport  Port=2
  coeffIn : Inport  Port=3
  Data Type Duplicate : DataTypeDuplicate
  Data Type Conversion : DataTypeConversion
  For Each Subsystem : Subsystem  TreatAsAtomicUnit=on
  Reshape : Reshape
  Reshape1 : Reshape  OutputDimensionality=Row vector (2-D)
  Reshape2 : Reshape
  Reshape3 : Reshape
  Selector : Selector  InputPortWidth=4  IndexOptions=Index vector (dialog)  Indices=1  OutputSizes=1
  dataOut : Outport
  validOut : Outport  Port=2
  wires:
  coeffIn/1 -> Reshape3/1
  dataIn/1 -> Reshape2/1
  validIn/1 -> For Each Subsystem/2(validIn)
  For Each Subsystem/2(validOut) -> Reshape/1
  For Each Subsystem/1(dataOut) -> Data Type Conversion/1
  Selector/1 -> validOut/1
  Reshape/1 -> Selector/1
  Reshape1/1 -> dataOut/1
  Reshape2/1 -> Data Type Duplicate/1, For Each Subsystem/1(dataIn)
  Reshape3/1 -> For Each Subsystem/3(coeffIn)
  Data Type Conversion/1 -> Data Type Duplicate/2, Reshape1/1

== system TxSteering_RxMVDR_4x4_HDL_IQ/DUT/ConcatADCChannels/To Data Bus ==
  data : Inport
  valid : Inport  Port=2
  Bus Creator : BusCreator  Inputs=2
  bus : Outport  VectorParamsAs1DForOutWhenUnconnected=off
  wires:
  Bus Creator/1 -> bus/1
  data/1 -> Bus Creator/1  "data"
  valid/1 -> Bus Creator/2  "valid"

== system TxSteering_RxMVDR_4x4_HDL_IQ/DUT/MVDR/Compute Weight Vector ==
  covarianceMatrix : Inport
  validIn : Inport  Port=2
  steeringVector : Inport  Port=3
  Data Type Conversion1 : DataTypeConversion  OutDataTypeStr=matrixdivin_dt
  Data Type Conversion2 : DataTypeConversion  OutDataTypeStr=matrixdivin_dt
  Data Type Conversion3 : DataTypeConversion  OutDataTypeStr=matrixdivout_dt
  Delay : Delay  DelayLength=1
  Logical Operator : Logic  IconShape=distinctive  AllPortsSameDT=off  OutDataTypeStr=boolean
  Matrix Left Divide : Subsystem  Variant=on  VariantControlMode=Label  LabelModeActiveChoice=HDL
  To Workspace : ToWorkspace  VariableName=sim_ready  SampleTime=-1
      settings: Save2DSignal=2-D array (concatenate along first dimension)
  w : Outport
  validOut : Outport  Port=2
  wires:
  covarianceMatrix/1 -> Data Type Conversion1/1
  steeringVector/1 -> Data Type Conversion2/1
  Data Type Conversion3/1 -> w/1
  Data Type Conversion1/1 -> Matrix Left Divide/1(A)
  Data Type Conversion2/1 -> Matrix Left Divide/2(B)
  Matrix Left Divide/2(validOut) -> validOut/1
  Matrix Left Divide/3(ready) -> Delay/1, To Workspace/1
  Matrix Left Divide/1(x) -> Data Type Conversion3/1
  validIn/1 -> Logical Operator/1
  Logical Operator/1 -> Matrix Left Divide/3(validIn)
  Delay/1 -> Logical Operator/2

== system TxSteering_RxMVDR_4x4_HDL_IQ/DUT/MVDR/Form Beam ==
  Bus Element In : Inport  PortName=DataBusIn  Element=data
  Bus Element In1 : Inport  PortName=DataBusIn  Element=valid
  w : Inport  Port=2
  Data Type Conversion : DataTypeConversion  OutDataTypeStr=output_dt
  Delay1 : Delay  DelayLength=6
  Delay2 : Delay
  Math Function2 : Math  Operator=conj  SaturateOnIntegerOverflow=on
  Parallel Complex Multiply : Subsystem  TreatAsAtomicUnit=on
  Reshape : Reshape
  Reshape1 : Reshape
  Tree Sum : Subsystem
  Bus Element Out : Outport  PortName=DataBusOut  Element=data
  Out Bus Element : Outport  PortName=DataBusOut  Element=valid
  wires:
  Bus Element In/1 -> Reshape1/1
  Parallel Complex Multiply/1(z) -> Tree Sum/1(In1)
  Tree Sum/1(Out1) -> Data Type Conversion/1
  Math Function2/1 -> Reshape/1
  w/1 -> Math Function2/1
  Reshape/1 -> Parallel Complex Multiply/2(z2)
  Reshape1/1 -> Parallel Complex Multiply/1(z1)
  Data Type Conversion/1 -> Bus Element Out/1
  Delay2/1 -> Out Bus Element/1
  Delay1/1 -> Delay2/1
  Bus Element In1/1 -> Delay1/1

== system TxSteering_RxMVDR_4x4_HDL_IQ/DUT/MVDR/Form Covariance Matrix ==
  note: Reshape the output of this block to 4x4
      | to produce the correct matrix structure:
      |
      | x1x'1
      | x1x'2
      | x1x'3
      | x1x'4
      |
      | x2x'1
      | x2x'2
      | x2x'3
      | x2x'4
      |
      | x3x'1
      | x3x'2
      | x3x'3
      | x3x'4
      |
      | x4x'1
      | x4x'2
      | x4x'3
      | x4x'4
  dataIn : Inport
  validIn : Inport  Port=2
  Conj : Math  Operator=conj
  Data Type Conversion : DataTypeConversion  OutDataTypeStr=covmat_dt
  Data Type Conversion1 : DataTypeConversion  OutDataTypeStr=adc_dt
  Delay : Delay  DelayLength=6
  Matrix Multiply Partitioned : Subsystem  TreatAsAtomicUnit=on
  Reshape : Reshape
  dataOut : Outport
  validOut : Outport  Port=2
  wires:
  validIn/1 -> Delay/1
  dataIn/1 -> Data Type Conversion1/1
  Reshape/1 -> Conj/1, Matrix Multiply Partitioned/1(x)  "x"
  Matrix Multiply Partitioned/1(C) -> Data Type Conversion/1  "x * x'"
  Delay/1 -> validOut/1
  Conj/1 -> Matrix Multiply Partitioned/2(x_conj)
  Data Type Conversion1/1 -> Reshape/1
  Data Type Conversion/1 -> dataOut/1

== system TxSteering_RxMVDR_4x4_HDL_IQ/DUT/MVDR/From Data Bus ==
  bus : Inport
  Bus Selector : BusSelector  OutputSignals=data,valid
  data : Outport  VectorParamsAs1DForOutWhenUnconnected=off
  valid : Outport  Port=2  VectorParamsAs1DForOutWhenUnconnected=off
  wires:
  Bus Selector/2 -> valid/1  "<valid>"
  Bus Selector/1 -> data/1  "<data>"
  bus/1 -> Bus Selector/1

== system TxSteering_RxMVDR_4x4_HDL_IQ/DUT/MVDR/Moving Average ==
  note: Shift replaces gain by 1/sqrt(windowSize)
  dataIn : Inport
  validIn : Inport  Port=2
  Add : Sum  Inputs=++-  AccumDataTypeStr=movavg_accum_dt  OutDataTypeStr=Inherit: Same as accumulator
  Bit Shift : hdlsllib/Logic and Bit Operations/Bit Shift  mode=Shift Right Arithmetic  N=movavg_bitshift
  Data Type Conversion : DataTypeConversion  OutDataTypeStr=movavg_out_dt
  Delay : Delay  DelayLength=windowSize
  Delay{1..5} (5 alike) : Delay  DelayLength=1
  Wait for Running Sum Init : Subsystem
  dataOut : Outport
  validOut : Outport  Port=2
  wires:
  Bit Shift/1 -> Data Type Conversion/1
  Delay1/1 -> Bit Shift/1, Add/1
  Delay/1 -> Add/3
  Add/1 -> Delay1/1
  dataIn/1 -> Delay2/1
  validIn/1 -> Delay3/1
  Delay2/1 -> Delay/1, Add/2
  Delay4/1 -> dataOut/1
  Delay5/1 -> validOut/1
  Data Type Conversion/1 -> Delay4/1
  Delay3/1 -> Wait for Running Sum Init/1(In1)
  Wait for Running Sum Init/1(Out1) -> Delay5/1

== system TxSteering_RxMVDR_4x4_HDL_IQ/DUT/MVDR/Normalize Response ==
  note: This subsystem scales the weight vector to ensure unit gain in the target direction.
  wIn : Inport
  validIn : Inport  Port=2
  steeringVector : Inport  Port=3
  MVDR Weight Update : Subsystem
  Unit Delay Enabled Synchronous : hdlsllib/Discrete/Unit Delay Enabled Synchronous  InitialCondition=0.0  SampleTime=-1
      settings: SourceProductBaseCode=SL
  wOut : Outport
  wires:
  steeringVector/1 -> MVDR Weight Update/1(Steering Vector)
  wIn/1 -> MVDR Weight Update/2(x)
  MVDR Weight Update/1(w) -> Unit Delay Enabled Synchronous/1
  MVDR Weight Update/2(validOut) -> Unit Delay Enabled Synchronous/2
  Unit Delay Enabled Synchronous/1 -> wOut/1
  validIn/1 -> MVDR Weight Update/3(validIn)

== system TxSteering_RxMVDR_4x4_HDL_IQ/DUT/MVDR/Subsystem ==
  BypassEn : Inport
  Bypass_Input : Inport  Port=2
  MVDR_Input : Inport  Port=3
  Delay : Delay  DelayLength=1
  Delay1 : Delay  DelayLength=1
  Delay2 : Delay  DelayLength=1
  RepackageInput : Subsystem
  RepackageMVDR : Subsystem
  Switch : Switch  Criteria=u2 > Threshold
  DataOut : Outport
  wires:
  BypassEn/1 -> Delay2/1
  RepackageMVDR/1(Out1) -> Switch/3
  MVDR_Input/1 -> Delay1/1
  Bypass_Input/1 -> Delay/1
  RepackageInput/1(Out1) -> Switch/1
  Switch/1 -> DataOut/1
  Delay/1 -> RepackageInput/1(In1)
  Delay1/1 -> RepackageMVDR/1(In3)
  Delay2/1 -> Switch/2

== system TxSteering_RxMVDR_4x4_HDL_IQ/DUT/Rx Data Capture/AXI4-Lite Initial Value ==
  In1 : Inport
  Compare To Zero : simulink/Logic and Bit Operations/Compare To Zero  relop=~=  OutDataTypeStr=boolean
  Logical Operator : Logic  Operator=OR  IconShape=distinctive  AllPortsSameDT=off  OutDataTypeStr=boolean
  Set_Latch : Subsystem
  Unit Delay Enabled Synchronous : hdlsllib/Discrete/Unit Delay Enabled Synchronous  InitialCondition=x0  SampleTime=-1
      settings: SourceProductBaseCode=SL
  Out1 : Outport  VectorParamsAs1DForOutWhenUnconnected=off
  wires:
  In1/1 -> Unit Delay Enabled Synchronous/1, Compare To Zero/1
  Logical Operator/1 -> Unit Delay Enabled Synchronous/2
  Compare To Zero/1 -> Logical Operator/1, Set_Latch/1(S)
  Set_Latch/1(Q) -> Logical Operator/2
  Unit Delay Enabled Synchronous/1 -> Out1/1

== system TxSteering_RxMVDR_4x4_HDL_IQ/DUT/Rx Data Capture/AutoTrigger ==
  MaxCount : Inport
  SW_en : Inport  Port=2
  DataPushFrequency : hdlsllib/Sources/HDL Counter  CountType=Free running  CountInit=0  CountStep=1  CountMax=25  CountFromType=Initial value  CountFrom=0  CountResetPort=on  CountLoadPort=off  CountEnbPort=on  CountDirPort=off  CountDataType=Unsigned  CountWordLen=32  CountFracLen=0  CountSampTime=1
  Detect Increase : simulink/Logic and Bit Operations/Detect Increase  vinit=0.0  OutDataTypeStr=boolean
  Relational Operator : RelationalOperator  Operator===  OutDataTypeStr=boolean  RndMeth=Simplest
  Trig : Outport  VectorParamsAs1DForOutWhenUnconnected=off
  wires:
  Relational Operator/1 -> DataPushFrequency/1, Detect Increase/1
  DataPushFrequency/1 -> Relational Operator/2  "DataPushFrequencyCount"
  Detect Increase/1 -> Trig/1
  SW_en/1 -> DataPushFrequency/2
  MaxCount/1 -> Relational Operator/1

== system TxSteering_RxMVDR_4x4_HDL_IQ/DUT/Rx Data Capture/EnableConsecutiveFrames ==
  note: Pause counter when experiencing backpressure
  note: Handle edge-case if we're at the
      | max counter value and we have back-pressure, do not reset
      | just yet. Wait for back pressure to clear then a reset can be applied
  note: Count to N samples specified by AXI-lite consec frames input
  Trigger : Inport
  ConsecFrames : Inport  Port=2
  BackPressureCounterEn : Inport  Port=3
  Compare To Zero1 : simulink/Logic and Bit Operations/Compare To Zero  relop=~=  OutDataTypeStr=boolean
  Data Type Conversion : DataTypeConversion  OutDataTypeStr=boolean
  DefaultConsecFrames : Constant  Value=1024*5  OutDataTypeStr=uint32  SampleTime=-1
  Delay : Delay  DelayLength=1
  Detect Increase : simulink/Logic and Bit Operations/Detect Increase  vinit=0.0  OutDataTypeStr=boolean
  HDL Counter : hdlsllib/Sources/HDL Counter  CountType=Free running  CountInit=0  CountStep=1  CountMax=25  CountFromType=Initial value  CountFrom=0  CountResetPort=on  CountLoadPort=off  CountEnbPort=on  CountDirPort=off  CountDataType=Unsigned  CountWordLen=32  CountFracLen=0  CountSampTime=1
  Logical Operator : Logic  IconShape=distinctive  AllPortsSameDT=off  OutDataTypeStr=boolean
  Logical Operator1 : Logic  IconShape=distinctive  AllPortsSameDT=off  OutDataTypeStr=boolean
  Logical Operator2 : Logic  IconShape=distinctive  AllPortsSameDT=off  OutDataTypeStr=boolean
  Relational Operator : RelationalOperator  Operator===  OutDataTypeStr=boolean  RndMeth=Simplest
  Signal Specification : SignalSpecification  OutDataTypeStr=boolean  Dimensions=1
  Switch : Switch  Criteria=u2 ~= 0
  sr_latch : Subsystem
  DataCaptureEn : Outport  VectorParamsAs1DForOutWhenUnconnected=off
  wires:
  Signal Specification/1 -> DataCaptureEn/1  "DataCaptureEn"
  Detect Increase/1 -> sr_latch/1(S)
  sr_latch/1(Q) -> Logical Operator/1
  HDL Counter/1 -> Relational Operator/1, Data Type Conversion/1  "ValidCounter"
  Trigger/1 -> Detect Increase/1
  ConsecFrames/1 -> Switch/1, Compare To Zero1/1
  Compare To Zero1/1 -> Switch/2
  Switch/1 -> Delay/1
  DefaultConsecFrames/1 -> Switch/3
  Logical Operator/1 -> HDL Counter/2  "En"
  Data Type Conversion/1 -> Logical Operator1/1
  Logical Operator1/1 -> Signal Specification/1
  Relational Operator/1 -> Logical Operator2/1, sr_latch/2(R)  "EndOfFrame"
  BackPressureCounterEn/1 -> Logical Operator1/2, Logical Operator2/2, Logical Operator/2
  Logical Operator2/1 -> HDL Counter/1  "RstCount"
  Delay/1 -> Relational Operator/2

== system TxSteering_RxMVDR_4x4_HDL_IQ/DUT/Rx Data Capture/Stream FIFO  ==
  TReady : Inport
  TData : Inport  Port=2
  TValid : Inport  Port=3
  TriggerCapture : Inport  Port=4
  StreamEn : Inport  Port=5
  Display : Display
  Logical Operator : Logic  AllPortsSameDT=off  OutDataTypeStr=boolean
  Logical Operator1 : Logic  IconShape=distinctive  AllPortsSameDT=off  OutDataTypeStr=boolean
  Logical Operator4 : Logic  Operator=NOT  IconShape=distinctive  AllPortsSameDT=off  OutDataTypeStr=boolean
  Logical Operator5 : Logic  IconShape=distinctive  AllPortsSameDT=off  OutDataTypeStr=boolean
  Logical Operator6 : Logic  Operator=NOT  IconShape=distinctive  AllPortsSameDT=off  OutDataTypeStr=boolean
  Logical Operator7 : Logic  IconShape=distinctive  AllPortsSameDT=off  OutDataTypeStr=boolean
  hdl_fwft_fifo : Subsystem  mask{FIFO_DEPTH=1024*10, AFULL_THRESH=10}
      mask prompts: FIFO_DEPTH "FIFO Depth"; AFULL_THRESH "Almost Full Threshold"
      mask init:
      | FIFO_CNT_BITS=ceil(log2(FIFO_DEPTH+1+3));
  TDataOut : Outport  VectorParamsAs1DForOutWhenUnconnected=off
  ValidOut : Outport  Port=2  VectorParamsAs1DForOutWhenUnconnected=off
  Num : Outport  Port=3  VectorParamsAs1DForOutWhenUnconnected=off
  Full : Outport  Port=4  VectorParamsAs1DForOutWhenUnconnected=off
  AFull : Outport  Port=5  VectorParamsAs1DForOutWhenUnconnected=off
  wires:
  TValid/1 -> Logical Operator/1
  Logical Operator6/1 -> Logical Operator7/1
  Logical Operator4/1 -> Logical Operator5/2
  Logical Operator5/1 -> Logical Operator1/1, hdl_fwft_fifo/3(rd_ack)
  Logical Operator7/1 -> hdl_fwft_fifo/2(push)
  TReady/1 -> Logical Operator5/1
  hdl_fwft_fifo/5(afull) -> AFull/1, Logical Operator6/1
  hdl_fwft_fifo/4(full) -> Full/1
  Logical Operator/1 -> Logical Operator7/2
  hdl_fwft_fifo/2(empty) -> Logical Operator4/1
  hdl_fwft_fifo/3(num) -> Display/1, Num/1
  TriggerCapture/1 -> Logical Operator/2
  TData/1 -> hdl_fwft_fifo/1(data_i)
  hdl_fwft_fifo/1(data_o) -> TDataOut/1
  Logical Operator1/1 -> ValidOut/1
  StreamEn/1 -> Logical Operator1/2

== system TxSteering_RxMVDR_4x4_HDL_IQ/DUT/Tx Signal Generation/Combine Channels ==
  dataIn : Inport
  validIn : Inport  Port=2
  Add : Sum
  Bit Shift : hdlsllib/Logic and Bit Operations/Bit Shift  mode=Shift Right Arithmetic  N=1
  Data Type Conversion : DataTypeConversion  OutDataTypeStr=int16
  Delay{,1..4} (5 alike) : Delay  DelayLength=1
  Selector : Selector  InputPortWidth=2  IndexOptions=Index vector (dialog)  Indices=1  OutputSizes=1
  Selector1 : Selector  InputPortWidth=8  IndexOptions=Index vector (dialog)  Indices=1:4  OutputSizes=1
  Selector2 : Selector  InputPortWidth=8  IndexOptions=Index vector (dialog)  Indices=5:8  OutputSizes=1
  dataOut : Outport
  validOut : Outport  Port=2
  wires:
  Bit Shift/1 -> Data Type Conversion/1
  dataIn/1 -> Selector2/1, Selector1/1
  validIn/1 -> Selector/1
  Selector/1 -> Delay3/1
  Selector2/1 -> Delay1/1
  Selector1/1 -> Delay/1
  Delay/1 -> Add/1
  Delay1/1 -> Add/2
  Delay2/1 -> Bit Shift/1
  Add/1 -> Delay2/1
  Data Type Conversion/1 -> dataOut/1
  Delay3/1 -> Delay4/1
  Delay4/1 -> validOut/1
